simulink model "complete_model1.0"  (R2022b)
settings: Solver=ode15s  StartTime=0.0  StopTime=10.0  RelTol=1e-3
undefined symbols (not defined in the file): g, Inertia
libraries: sharedutil x2, Aerodynamics_library x1, Atmospheric_final x1, propulsion x1
settings Model: Creator=Dell  LastModifiedBy=Dell
settings DebuggingCC: IntegerSaturationMsg=none

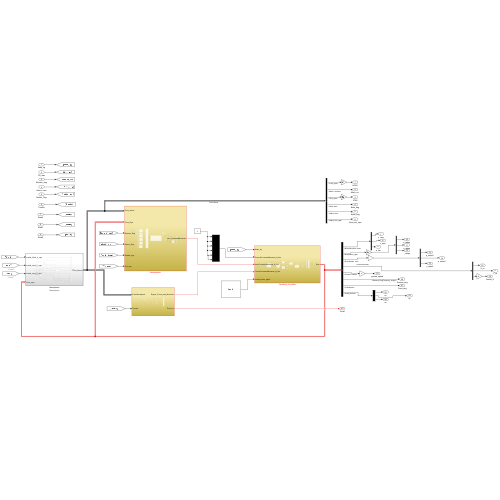
[thumbnail: Simulink's stored preview of the top-level diagram]
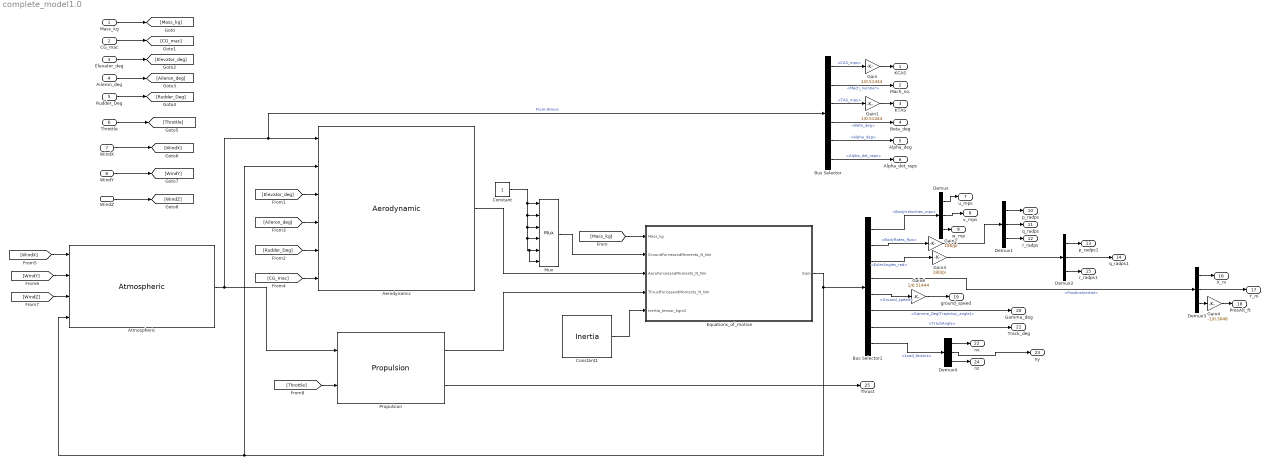
== system complete_model1.0 ==
  Mass_kg : Inport
  CG_mac : Inport  Port=2
  Elevator_deg : Inport  Port=3
  Aileron_deg : Inport  Port=4
  Rudder_Deg : Inport  Port=5
  Throttle : Inport  Port=6
  WindX : Inport  Port=7
  WindY : Inport  Port=8
  WindZ : Inport  Port=9
  Aerodynamic : Aerodynamics_library/Aerodynamic  SystemSampleTime=-1  VariantActivationTime=update diagram  Latency=0  AutoFrameSizeCalculation=off
  Atmospheric : Atmospheric_final/Atmospheric  Description=Atmospheric  SystemSampleTime=-1  VariantActivationTime=update diagram  Latency=0  AutoFrameSizeCalculation=off
      settings: AttributesFormatString=Atmospheric
  Bus Selector : BusSelector  OutputSignals=CAS_mps,Mach_number,TAS_mps,Beta_deg,Alpha_deg,Alpha_dot_raps
  Bus Selector1 : BusSelector  OutputSignals=BodyVelocities_mps,BodyRates_Rps,EulerAngles_rad,PositionInertial,Ground_speed,Gamma_Deg(Trajectoy_angle),TrackAngle,Load_factors
  Constant : Constant
  Constant1 : Constant  Value=Inertia
  Demux{,1..4} (5 alike) : Demux  Outputs=3
  Equations_of_motion : Subsystem
      settings: LibrarySourceBlock=Equations_of_motion_block/Equations_of_motion
  Gain : Gain  Gain=1/0.51444
  Gain1 : Gain  Gain=1/0.51444
  Gain2 : Gain  Gain=180/pi
  Gain3 : Gain  Gain=180/pi
  Gain4 : Gain  Gain=-1/0.3048
  Gain6 : Gain  Gain=1/0.51444
  Mux : Mux  Inputs=6
  Propulsion : propulsion/Propulsion  SystemSampleTime=-1  VariantActivationTime=update diagram  Latency=0  AutoFrameSizeCalculation=off
  KCAS : Outport
  Mach_no. : Outport  Port=2
  KTAS : Outport  Port=3
  Beta_deg : Outport  Port=4
  Alpha_deg : Outport  Port=5
  Alpha_dot_raps : Outport  Port=6
  u_mps : Outport  Port=7
  v_mps : Outport  Port=8
  w_mp : Outport  Port=9
  p_radps : Outport  Port=10
  q_radps : Outport  Port=11
  r_radps : Outport  Port=12
  p_radps1 : Outport  Port=13
  q_radps1 : Outport  Port=14
  r_radps1 : Outport  Port=15
  X_m : Outport  Port=16
  Y_m : Outport  Port=17
  PresAlt_ft : Outport  Port=18
  ground_speed : Outport  Port=19
  Gamma_deg : Outport  Port=20
  Track_deg : Outport  Port=21
  nx : Outport  Port=22
  ny : Outport  Port=23
  nz : Outport  Port=24
  Thrust : Outport  Port=25
  wires:
  Atmospheric/1 -> Propulsion/1, Bus Selector/1, Aerodynamic/1  "From-Atmos"
  Aerodynamic/1 -> Equations_of_motion/3(AeroForcesandMoments_N_Nm)
  Propulsion/1 -> Equations_of_motion/4(ThrustForcesandMoments_N_Nm)
  Equations_of_motion/1(Eqm) -> Bus Selector1/1, Aerodynamic/2, Atmospheric/4
  Constant/1 -> Mux/6, Mux/5, Mux/4, Mux/3, Mux/2, Mux/1
  Mux/1 -> Equations_of_motion/2(GroundForcesandMoments_N_Nm)
  Constant1/1 -> Equations_of_motion/5(Inertia_tensor_kgm2)
  Mass_kg/1 -> [Mass_kg]
  WindX/1 -> [WindX]
  Throttle/1 -> [Throttle]
  Rudder_Deg/1 -> [Rudder_Deg]
  Aileron_deg/1 -> [Aileron_deg]
  Elevator_deg/1 -> [Elevator_deg]
  CG_mac/1 -> [CG_mac]
  WindY/1 -> [WindY]
  WindZ/1 -> [WindZ]
  [Elevator_deg] -> Aerodynamic/3
  [Rudder_Deg] -> Aerodynamic/5
  [Aileron_deg] -> Aerodynamic/4
  [CG_mac] -> Aerodynamic/6
  [WindX] -> Atmospheric/1
  [WindY] -> Atmospheric/2
  [WindZ] -> Atmospheric/3
  [Throttle] -> Propulsion/2
  [Mass_kg] -> Equations_of_motion/1(Mass_kg)
  Propulsion/2 -> Thrust/1
  Bus Selector1/8 -> Demux4/1  "<Load_factors>"
  Bus Selector1/7 -> Track_deg/1  "<TrackAngle>"
  Bus Selector1/6 -> Gamma_deg/1  "<Gamma_Deg(Trajectoy_angle)>"
  Bus Selector1/5 -> Gain6/1  "<Ground_speed>"
  Bus Selector1/4 -> Demux3/1  "<PositionInertial>"
  Bus Selector1/3 -> Gain3/1  "<EulerAngles_rad>"
  Bus Selector1/1 -> Demux/1  "<BodyVelocities_mps>"
  Bus Selector/6 -> Alpha_dot_raps/1  "<Alpha_dot_raps>"
  Bus Selector/5 -> Alpha_deg/1  "<Alpha_deg>"
  Bus Selector/4 -> Beta_deg/1  "<Beta_deg>"
  Bus Selector/3 -> Gain1/1  "<TAS_mps>"
  Bus Selector/2 -> Mach_no./1  "<Mach_number>"
  Bus Selector/1 -> Gain/1  "<CAS_mps>"
  Gain/1 -> KCAS/1
  Gain1/1 -> KTAS/1
  Demux/3 -> w_mp/1
  Demux/2 -> v_mps/1
  Demux/1 -> u_mps/1
  Demux1/2 -> q_radps/1
  Demux1/3 -> r_radps/1
  Demux1/1 -> p_radps/1
  Bus Selector1/2 -> Gain2/1  "<BodyRates_Rps>"
  Gain2/1 -> Demux1/1
  Demux2/2 -> q_radps1/1
  Demux2/3 -> r_radps1/1
  Demux2/1 -> p_radps1/1
  Gain3/1 -> Demux2/1
  Demux3/2 -> Y_m/1
  Demux3/3 -> Gain4/1
  Demux3/1 -> X_m/1
  Gain4/1 -> PresAlt_ft/1
  Gain6/1 -> ground_speed/1
  Demux4/2 -> ny/1
  Demux4/1 -> nx/1
  Demux4/3 -> nz/1

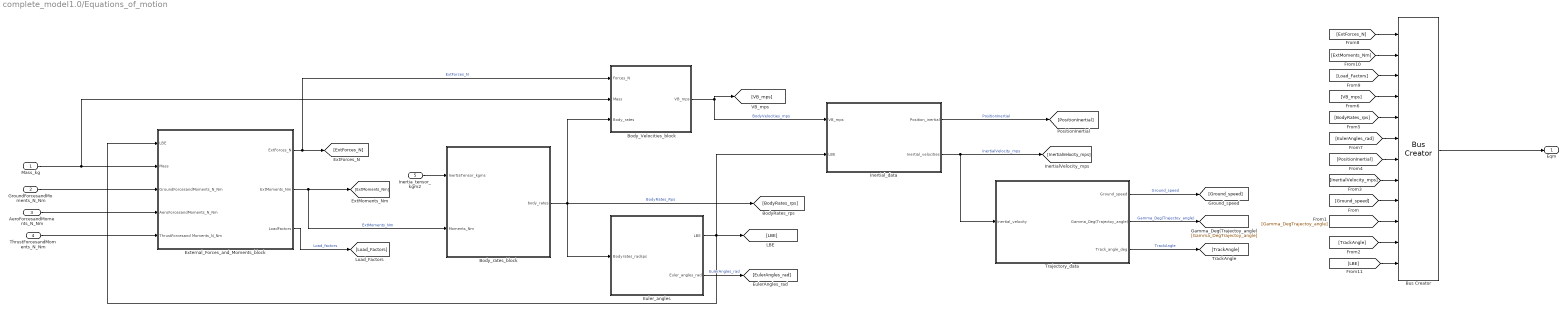
== system complete_model1.0/Equations_of_motion ==
  Mass_kg : Inport
  GroundForcesandMoments_N_Nm : Inport  Port=2
  AeroForcesandMoments_N_Nm : Inport  Port=3
  ThrustForcesandMoments_N_Nm : Inport  Port=4
  Inertia_tensor_kgm2 : Inport  Port=5
  Body_Velocities_block : Subsystem
  Body_rates_block : Subsystem
  Bus Creator : BusCreator  Inputs=12
  Euler_angles : Subsystem
  External_Forces_and_Moments_block : Subsystem
  Inertial_data : Subsystem
  Trajectory_data : Subsystem
  Eqm : Outport
  wires:
  [Load_Factors] -> Bus Creator/3
  [Ground_speed] -> Bus Creator/9
  [TrackAngle] -> Bus Creator/11
  [VB_mps] -> Bus Creator/4
  [ExtMoments_Nm] -> Bus Creator/2
  Trajectory_data/3(Track_angle_deg) -> [TrackAngle]  "TrackAngle"
  Euler_angles/2(Euler_angles_rad) -> [EulerAngles_rad]  "EulerAngles_rad"
  Trajectory_data/1(Ground_speed) -> [Ground_speed]  "Ground_speed"
  [EulerAngles_rad] -> Bus Creator/6
  [Gamma_DegTrajectoy_angle] -> Bus Creator/10
  Bus Creator/1 -> Eqm/1
  Trajectory_data/2(Gamma_Deg(Trajectoy_angle)) -> [Gamma_DegTrajectoy_angle]  "Gamma_Deg(Trajectoy_angle)"
  Euler_angles/1(LBE) -> Inertial_data/2(LBE), [LBE], External_Forces_and_Moments_block/1(LBE)
  [BodyRates_rps] -> Bus Creator/5
  External_Forces_and_Moments_block/3(LoadFactors) -> [Load_Factors]  "Load_factors"
  Inertial_data/1(Position_inertial) -> [PositionInertial]  "PositionInertial"
  Body_Velocities_block/1(VB_mps) -> [VB_mps], Inertial_data/1(VB_mps)  "BodyVelocities_mps"
  Body_rates_block/1(body_rates) -> Body_Velocities_block/3(Body_rates), [BodyRates_rps], Euler_angles/1(Bodyrates_radsps)  "BodyRates_Rps"
  ThrustForcesandMoments_N_Nm/1 -> External_Forces_and_Moments_block/5(ThrustForcesand Moments_N_Nm)
  AeroForcesandMoments_N_Nm/1 -> External_Forces_and_Moments_block/4(AeroForcesandMoments_N_Nm)
  GroundForcesandMoments_N_Nm/1 -> External_Forces_and_Moments_block/3(GroundForcesandMoments_N_Nm)
  [ExtForces_N] -> Bus Creator/1
  [InertialVelocity_mps] -> Bus Creator/8
  Inertia_tensor_kgm2/1 -> Body_rates_block/1(InertiaTensor_kgms)
  External_Forces_and_Moments_block/2(ExtMoments_Nm) -> [ExtMoments_Nm], Body_rates_block/2(Moments_Nm)  "ExtMoments_Nm"
  Mass_kg/1 -> External_Forces_and_Moments_block/2(Mass), Body_Velocities_block/2(Mass)
  [PositionInertial] -> Bus Creator/7
  Inertial_data/2(Inertial_velocities) -> Trajectory_data/1(Inertial_velocity), [InertialVelocity_mps]  "InertialVelocity_mps"
  External_Forces_and_Moments_block/1(ExtForces_N) -> [ExtForces_N], Body_Velocities_block/1(Forces_N)  "ExtForces_N"
  [LBE] -> Bus Creator/12

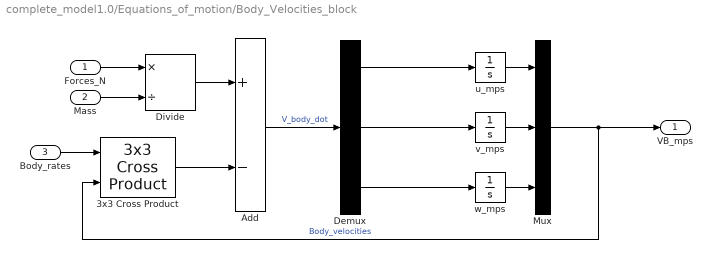
== system complete_model1.0/Equations_of_motion/Body_Velocities_block ==
  Forces_N : Inport
  Mass : Inport  Port=2
  Body_rates : Inport  Port=3
  3x3 Cross Product : sharedutil/3x3 Cross Product  aMode=aMode
      settings: LibrarySourceBlock=aerolibutil/3x3 Cross Product
  Add : Sum  Inputs=+-
  Demux : Demux  Outputs=3
  Divide : Product  Inputs=*/
  Mux : Mux  Inputs=3
  u_mps : Integrator  ContinuousStateAttributes='u_mps'
  v_mps : Integrator  ContinuousStateAttributes='v_mps'
  w_mps : Integrator  ContinuousStateAttributes='w_mps'
  VB_mps : Outport
  wires:
  Forces_N/1 -> Divide/1
  Demux/2 -> v_mps/1
  Divide/1 -> Add/1
  Demux/1 -> u_mps/1
  u_mps/1 -> Mux/1
  w_mps/1 -> Mux/3
  Mux/1 -> 3x3 Cross Product/2, VB_mps/1  "Body_velocities"
  v_mps/1 -> Mux/2
  Add/1 -> Demux/1  "V_body_dot"
  Mass/1 -> Divide/2
  Demux/3 -> w_mps/1
  Body_rates/1 -> 3x3 Cross Product/1
  3x3 Cross Product/1 -> Add/2

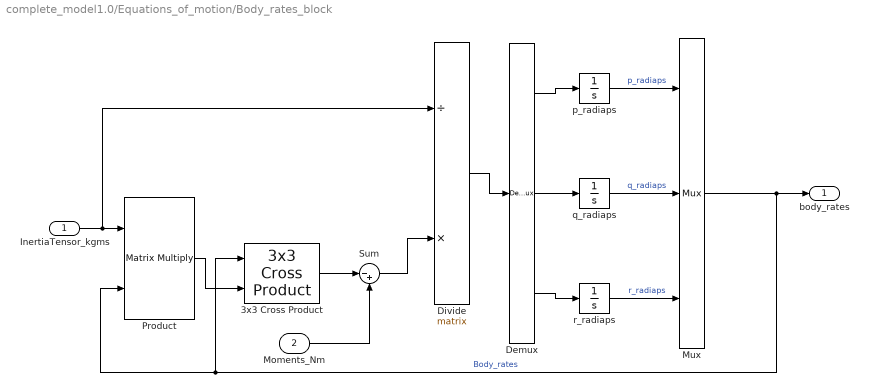
== system complete_model1.0/Equations_of_motion/Body_rates_block ==
  InertiaTensor_kgms : Inport
  Moments_Nm : Inport  Port=2
  3x3 Cross Product : sharedutil/3x3 Cross Product  aMode=aMode
      settings: LibrarySourceBlock=aerolibutil/3x3 Cross Product
  Demux : Demux  Outputs=3
  Divide : Product  Inputs=/*  Multiplication=Matrix(*)
  Mux : Mux  Inputs=3
  Product : Product  Multiplication=Matrix(*)
  Sum : Sum  Inputs=|-+
  p_radiaps : Integrator  ContinuousStateAttributes='p_radiaps'
  q_radiaps : Integrator  ContinuousStateAttributes='q_radiaps'
  r_radiaps : Integrator  ContinuousStateAttributes='r_radiaps'
  body_rates : Outport
  wires:
  InertiaTensor_kgms/1 -> Product/1, Divide/1
  Demux/3 -> r_radiaps/1
  p_radiaps/1 -> Mux/1  "p_radiaps"
  q_radiaps/1 -> Mux/2  "q_radiaps"
  Demux/2 -> q_radiaps/1
  Divide/1 -> Demux/1
  Demux/1 -> p_radiaps/1
  Mux/1 -> 3x3 Cross Product/1, Product/2, body_rates/1  "Body_rates"
  r_radiaps/1 -> Mux/3  "r_radiaps"
  Product/1 -> 3x3 Cross Product/2
  3x3 Cross Product/1 -> Sum/1
  Moments_Nm/1 -> Sum/2
  Sum/1 -> Divide/2

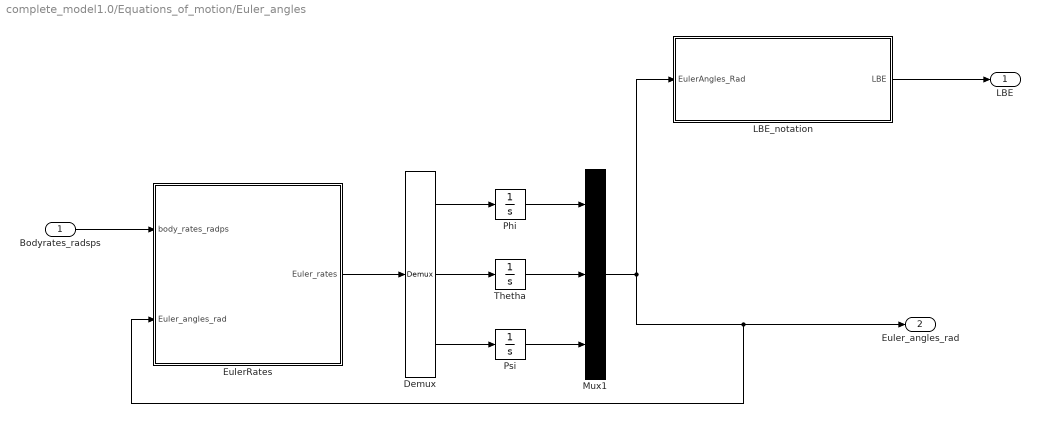
== system complete_model1.0/Equations_of_motion/Euler_angles ==
  Bodyrates_radsps : Inport
  Demux : Demux  Outputs=3
  EulerRates : Subsystem
  LBE_notation : Subsystem
  Mux1 : Mux  Inputs=3
  Phi : Integrator  ContinuousStateAttributes='Phi_ad'
  Psi : Integrator  ContinuousStateAttributes='Psi_rad'
  Thetha : Integrator  ContinuousStateAttributes='Theta_rad'
  LBE : Outport
  Euler_angles_rad : Outport  Port=2
  wires:
  Bodyrates_radsps/1 -> EulerRates/1(body_rates_radps)
  LBE_notation/1(LBE) -> LBE/1
  Demux/3 -> Psi/1
  EulerRates/1(Euler_rates) -> Demux/1
  Psi/1 -> Mux1/3
  Demux/1 -> Phi/1
  Thetha/1 -> Mux1/2
  Demux/2 -> Thetha/1
  Mux1/1 -> LBE_notation/1(EulerAngles_Rad), Euler_angles_rad/1, EulerRates/2(Euler_angles_rad)
  Phi/1 -> Mux1/1

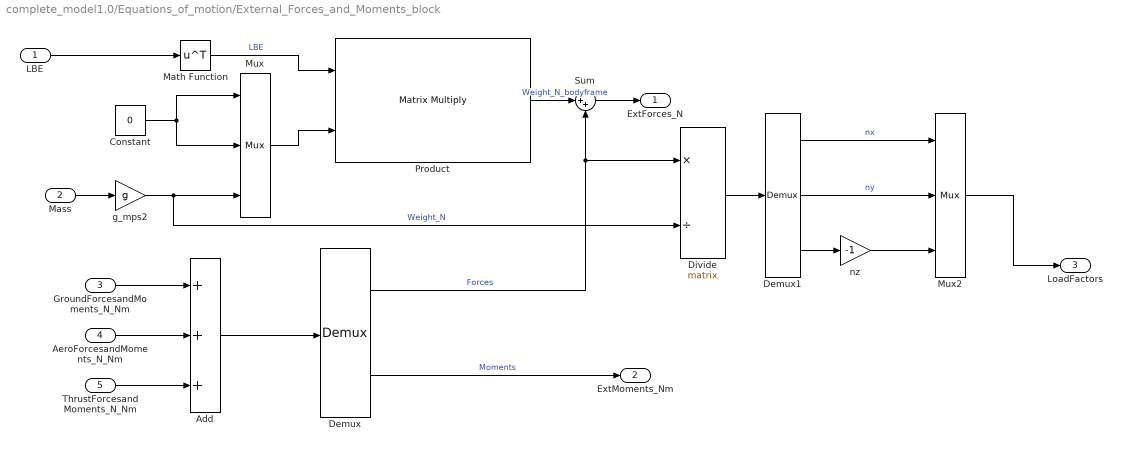
== system complete_model1.0/Equations_of_motion/External_Forces_and_Moments_block ==
  LBE : Inport
  Mass : Inport  Port=2
  GroundForcesandMoments_N_Nm : Inport  Port=3
  AeroForcesandMoments_N_Nm : Inport  Port=4
  ThrustForcesand Moments_N_Nm : Inport  Port=5
  Add : Sum  Inputs=+++
  Constant : Constant  Value=0
  Demux : Demux  Outputs=2
  Demux1 : Demux  Outputs=3
  Divide : Product  Inputs=*/  Multiplication=Matrix(*)
  Math Function : Math  Operator=transpose
  Mux : Mux  Inputs=3
  Mux2 : Mux  Inputs=3
  Product : Product  Multiplication=Matrix(*)
  Sum : Sum  Inputs=|++
  g_mps2 : Gain  Gain=g
  nz : Gain  Gain=-1
  ExtForces_N : Outport
  ExtMoments_Nm : Outport  Port=2
  LoadFactors : Outport  Port=3
  wires:
  LBE/1 -> Math Function/1
  Mux2/1 -> LoadFactors/1
  AeroForcesandMoments_N_Nm/1 -> Add/2
  GroundForcesandMoments_N_Nm/1 -> Add/1
  Divide/1 -> Demux1/1
  Sum/1 -> ExtForces_N/1
  Demux1/1 -> Mux2/1  "nx"
  Mux/1 -> Product/2
  ThrustForcesand Moments_N_Nm/1 -> Add/3
  Product/1 -> Sum/1  "Weight_N_bodyframe"
  Math Function/1 -> Product/1  "LBE"
  Demux1/3 -> nz/1
  nz/1 -> Mux2/3
  Mass/1 -> g_mps2/1
  Constant/1 -> Mux/2, Mux/1
  Demux1/2 -> Mux2/2  "ny"
  Demux/2 -> ExtMoments_Nm/1  "Moments"
  Demux/1 -> Divide/1, Sum/2  "Forces"
  Add/1 -> Demux/1
  g_mps2/1 -> Divide/2, Mux/3  "Weight_N"

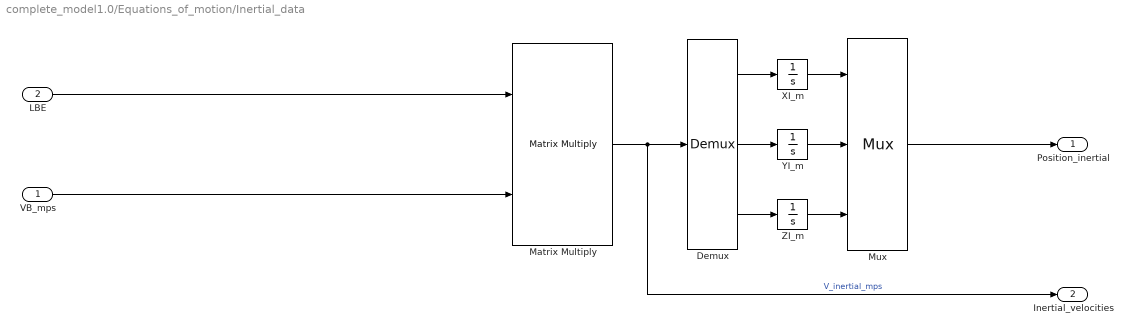
== system complete_model1.0/Equations_of_motion/Inertial_data ==
  VB_mps : Inport
  LBE : Inport  Port=2
  Demux : Demux  Outputs=3
  Matrix Multiply : Product  Multiplication=Matrix(*)
  Mux : Mux  Inputs=3
  XI_m : Integrator  ContinuousStateAttributes='XI_m'
  YI_m : Integrator  ContinuousStateAttributes='YI_m'
  ZI_m : Integrator  ContinuousStateAttributes='ZI_m'
  Position_inertial : Outport
  Inertial_velocities : Outport  Port=2
  wires:
  Matrix Multiply/1 -> Demux/1, Inertial_velocities/1  "V_inertial_mps"
  Demux/3 -> ZI_m/1
  XI_m/1 -> Mux/1
  YI_m/1 -> Mux/2
  ZI_m/1 -> Mux/3
  Mux/1 -> Position_inertial/1
  Demux/1 -> XI_m/1
  Demux/2 -> YI_m/1
  VB_mps/1 -> Matrix Multiply/2
  LBE/1 -> Matrix Multiply/1

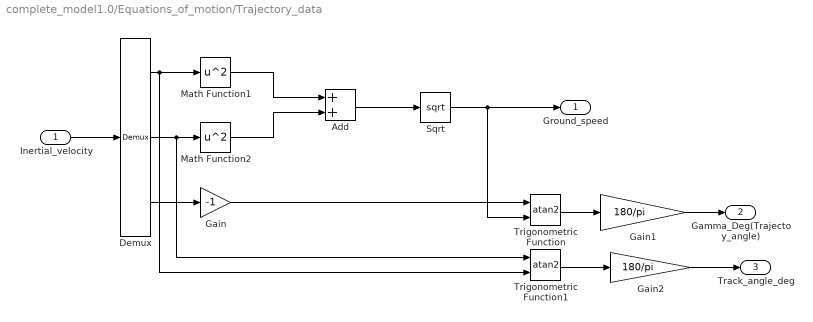
== system complete_model1.0/Equations_of_motion/Trajectory_data ==
  Inertial_velocity : Inport
  Add : Sum
  Demux : Demux  Outputs=3
  Gain : Gain  Gain=-1
  Gain1 : Gain  Gain=180/pi
  Gain2 : Gain  Gain=180/pi
  Math Function1 : Math  Operator=square
  Math Function2 : Math  Operator=square
  Sqrt : Sqrt
  Trigonometric Function : Trigonometry  Operator=atan2
  Trigonometric Function1 : Trigonometry  Operator=atan2
  Ground_speed : Outport
  Gamma_Deg(Trajectoy_angle) : Outport  Port=2
  Track_angle_deg : Outport  Port=3
  wires:
  Inertial_velocity/1 -> Demux/1
  Trigonometric Function1/1 -> Gain2/1
  Gain/1 -> Trigonometric Function/1
  Math Function2/1 -> Add/2
  Demux/2 -> Math Function2/1, Trigonometric Function1/1
  Gain2/1 -> Track_angle_deg/1
  Gain1/1 -> Gamma_Deg(Trajectoy_angle)/1
  Trigonometric Function/1 -> Gain1/1
  Math Function1/1 -> Add/1
  Sqrt/1 -> Ground_speed/1, Trigonometric Function/2
  Demux/1 -> Math Function1/1, Trigonometric Function1/2
  Demux/3 -> Gain/1
  Add/1 -> Sqrt/1

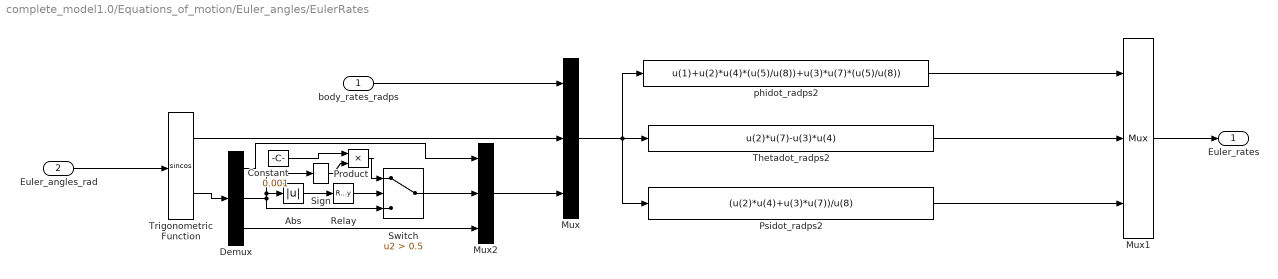
== system complete_model1.0/Equations_of_motion/Euler_angles/EulerRates ==
  body_rates_radps : Inport
  Euler_angles_rad : Inport  Port=2
  Abs : Abs  SaturateOnIntegerOverflow=off
  Constant : Constant  Value=0.001
  Demux : Demux  Outputs=3
  Mux : Mux  Inputs=3
  Mux1 : Mux  Inputs=3
  Mux2 : Mux  Inputs=3
  Product : Product
  Psidot_radps2 : MATLABFcn  MATLABFcn=(u(2)*u(4)+u(3)*u(7))/u(8)  OutputDimensions=1
  Relay : Relay  OnSwitchValue=0.001  OffSwitchValue=0  OnOutputValue=0  OffOutputValue=1
  Sign : Signum
  Switch : Switch  Criteria=u2 > Threshold  Threshold=0.5  SaturateOnIntegerOverflow=off  InputSameDT=off
  Thetadot_radps2 : MATLABFcn  MATLABFcn=u(2)*u(7)-u(3)*u(4)  OutputDimensions=1
  Trigonometric Function : Trigonometry  Operator=sincos
  phidot_radps2 : MATLABFcn  MATLABFcn=u(1)+u(2)*u(4)*(u(5)/u(8))+u(3)*u(7)*(u(5)/u(8))  OutputDimensions=1
  Euler_rates : Outport
  wires:
  Abs/1 -> Relay/1
  Sign/1 -> Product/2
  Product/1 -> Switch/1
  Demux/3 -> Mux2/3
  Constant/1 -> Product/1
  phidot_radps2/1 -> Mux1/1
  Mux1/1 -> Euler_rates/1
  Mux2/1 -> Mux/3
  Demux/1 -> Mux2/1
  Thetadot_radps2/1 -> Mux1/2
  Trigonometric Function/2 -> Demux/1
  Relay/1 -> Switch/2
  Switch/1 -> Mux2/2
  Mux/1 -> Psidot_radps2/1, Thetadot_radps2/1, phidot_radps2/1
  Trigonometric Function/1 -> Mux/2
  Demux/2 -> Switch/3, Abs/1, Sign/1
  body_rates_radps/1 -> Mux/1
  Euler_angles_rad/1 -> Trigonometric Function/1
  Psidot_radps2/1 -> Mux1/3

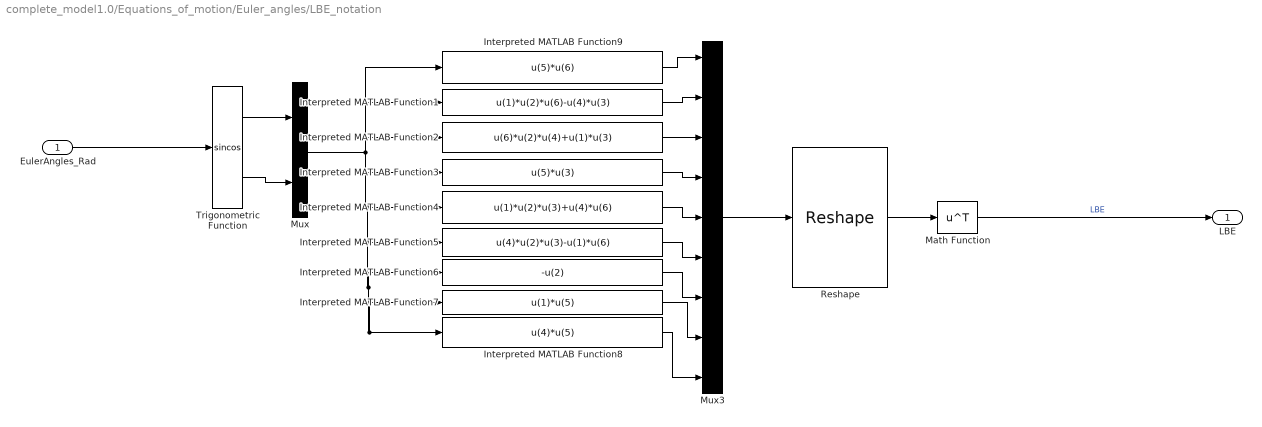
== system complete_model1.0/Equations_of_motion/Euler_angles/LBE_notation ==
  EulerAngles_Rad : Inport
  Interpreted MATLAB Function1 : MATLABFcn  MATLABFcn=u(1)*u(2)*u(6)-u(4)*u(3)  OutputDimensions=1
  Interpreted MATLAB Function2 : MATLABFcn  MATLABFcn=u(6)*u(2)*u(4)+u(1)*u(3)  OutputDimensions=1
  Interpreted MATLAB Function3 : MATLABFcn  MATLABFcn=u(5)*u(3)  OutputDimensions=1
  Interpreted MATLAB Function4 : MATLABFcn  MATLABFcn=u(1)*u(2)*u(3)+u(4)*u(6)  OutputDimensions=1
  Interpreted MATLAB Function5 : MATLABFcn  MATLABFcn=u(4)*u(2)*u(3)-u(1)*u(6)  OutputDimensions=1
  Interpreted MATLAB Function6 : MATLABFcn  MATLABFcn=-u(2)  OutputDimensions=1
  Interpreted MATLAB Function7 : MATLABFcn  MATLABFcn=u(1)*u(5)  OutputDimensions=1
  Interpreted MATLAB Function8 : MATLABFcn  MATLABFcn=u(4)*u(5)  OutputDimensions=1
  Interpreted MATLAB Function9 : MATLABFcn  MATLABFcn=u(5)*u(6)  OutputDimensions=1
  Math Function : Math  Operator=transpose
  Mux : Mux  Inputs=[3 3]
  Mux3 : Mux  Inputs=9
  Reshape : Reshape  OutputDimensionality=Customize  OutputDimensions=[3,3]
  Trigonometric Function : Trigonometry  Operator=sincos
  LBE : Outport
  wires:
  EulerAngles_Rad/1 -> Trigonometric Function/1
  Interpreted MATLAB Function9/1 -> Mux3/1
  Math Function/1 -> LBE/1  "LBE"
  Interpreted MATLAB Function3/1 -> Mux3/4
  Interpreted MATLAB Function2/1 -> Mux3/3
  Interpreted MATLAB Function5/1 -> Mux3/6
  Interpreted MATLAB Function7/1 -> Mux3/8
  Mux3/1 -> Reshape/1
  Interpreted MATLAB Function1/1 -> Mux3/2
  Interpreted MATLAB Function4/1 -> Mux3/5
  Reshape/1 -> Math Function/1
  Interpreted MATLAB Function8/1 -> Mux3/9
  Interpreted MATLAB Function6/1 -> Mux3/7
  Trigonometric Function/2 -> Mux/2
  Trigonometric Function/1 -> Mux/1
  Mux/1 -> Interpreted MATLAB Function3/1, Interpreted MATLAB Function4/1, Interpreted MATLAB Function5/1, Interpreted MATLAB Function6/1, Interpreted MATLAB Function7/1, Interpreted MATLAB Function8/1, Interpreted MATLAB Function1/1, Interpreted MATLAB Function9/1, Interpreted MATLAB Function2/1
